simulink model "Facies2022b"  (R2022b)
settings: Solver=VariableStepAuto  StartTime=0.0  StopTime=6  RelTol=1e-3
(part 2 of 2)

== matlab function Facies2022b/media ==
  data: u input; y output
function y = media(u)

y = mean(u);

== matlab function Facies2022b/media2 ==
  data: u input; y output
function y = media(u)

y = mean(u);

== matlab function Facies2022b/media1 ==
  data: u input; y output
function y = media(u)

y = mean(u);
